simulink model "quadcopter_model_c_EulerLagrange"  (Simulink 8.7)
settings: Solver=VariableStepAuto  StartTime=0.0  StopTime=2  RelTol=1e-3
undefined symbols (not defined in the file): A, g, I, m
settings Model: Creator=Daniel  LastModifiedBy=mgreiff
settings DataIOCC: SaveFormat=Dataset
settings DebuggingCC: UnderspecifiedInitializationDetection=Simplified  MergeDetectMultiDrivingBlocksExec=error  AllowSymbolicDim=off
settings HardwareCC: ProdBitPerPointer=64  ProdLargestAtomicFloat=Float  ProdIntDivRoundTo=Zero  ProdEndianess=LittleEndian  ProdWordSize=64  ProdHWDeviceType=Intel->x86-64 (Windows64)
settings GRTTargetCC: GeneratePreprocessorConditionals=Use local settings
settings ConfigComp: CovModelRefEnable=off

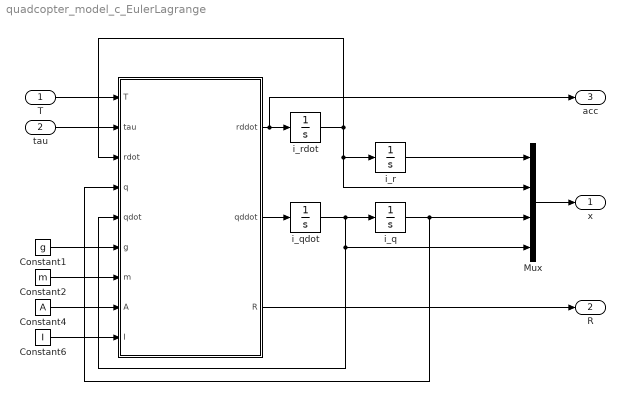
== system quadcopter_model_c_EulerLagrange ==
  T : Inport  PortDimensions=1
  tau : Inport  Port=2  PortDimensions=4
  " " : MATLAB Function  TreatAsAtomicUnit=on
  Constant1 : Constant  Value=g
  Constant2 : Constant  Value=m
  Constant4 : Constant  Value=A
  Constant6 : Constant  Value=I
  Mux : Mux
  i_q : Integrator  InitialCondition=[1 0 0 0]'
  i_qdot : Integrator  InitialCondition=[0; 0; 0; 0]
  i_r : Integrator  InitialCondition=[0 0 0]'
  i_rdot : Integrator  InitialCondition=[0; 0; 0]
  x : Outport
  R : Outport  Port=2
  acc : Outport  Port=3
  wires:
  " "/2(qddot) -> i_qdot/1
  " "/1(rddot) -> acc/1, i_rdot/1
  i_rdot/1 -> Mux/2, i_r/1, " "/3(rdot)
  i_qdot/1 -> " "/5(qdot), Mux/4, i_q/1
  i_r/1 -> Mux/1
  T/1 -> " "/1(T)
  Mux/1 -> x/1
  tau/1 -> " "/2(tau)
  i_q/1 -> " "/4(q), Mux/3
  Constant6/1 -> " "/9(I)
  Constant4/1 -> " "/8(A)
  Constant2/1 -> " "/7(m)
  Constant1/1 -> " "/6(g)
  " "/3(R) -> R/1

== matlab function   ==
  data: T input double; tau input double; rddot output double; rdot input double; q input double; qdot input double; qddot output double; g input double; m input double; A input double; I input double; R output double
function [ rddot,qddot,R] = quad_acceleration(T, tau, rdot, q, qdot, g, m, A, I)

    % T - total thrust in body coordinates
    % tau - torques in quaterion format
    
    a = 1;
    
    % normalize quaternion (?)
    q = q./sqrt(q'*q);
    
    qw = q(1); qx = q(2); qy = q(3); qz = q(4);
    
    % Gravity acceleration
    Ga = -g * [0; 0; 1];

    angM = [2*(qx*qz + qw*qy);
            2*(qy*qz - qw*qx);
            qw.^2 - qx.^2 - qy.^2 + qz.^2];
 
    Ta = T/m * angM;
    
    % Drag
    Aa = -1/m * diag(A) * rdot;    
    rddot = Ga + Ta + Aa;

    J = 4.*diag([a;I]);
    dJdq = 4.*diag([a;I]);
    C = -(1/2) .* dJdq;
    qddot = J\(tau - C * qdot);
    
    % Todo write out R matrix for visualisation if need be
    R = eye(3);
end
